simulink subsystem "accelerometer"  (R2024b)
settings: Solver=VariableStepAuto  StartTime=0.0  StopTime=10.0  RelTol=1e-3
undefined symbols (not defined in the file or in its folder): ACCEL_BIAS, ACCEL_COV, ACCEL_RANGE, ACCEL_RATE
settings Model: Creator=yevge  LastModifiedBy=Aiden Gaydos

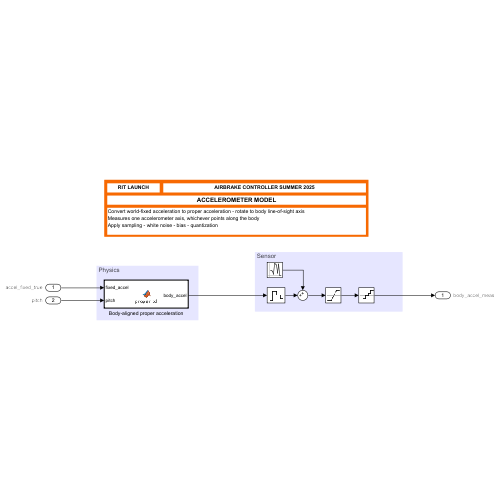
[thumbnail: Simulink's stored preview of the top-level diagram]
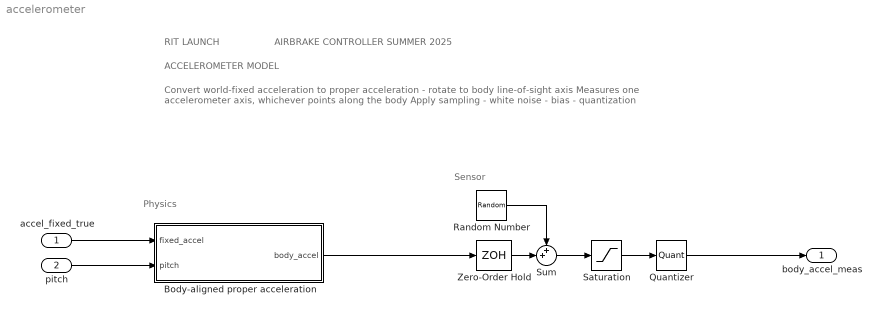
== system accelerometer ==
  note: Sensor
  note: Physics
  note: AIRBRAKE CONTROLLER SUMMER 2025
  note: RIT LAUNCH
  note: ACCELEROMETER MODEL
  note: Convert world-fixed acceleration to proper acceleration - rotate to body line-of-sight axis
      | Measures one accelerometer axis, whichever points along the body
      | Apply sampling - white noise - bias - quantization
  accel_fixed_true : Inport  Unit=m/s^2  PortDimensions=[2 1]
  pitch : Inport  Port=2  Unit=rad  PortDimensions=1
  Body-aligned proper acceleration : MATLAB Function  TreatAsAtomicUnit=on
  Quantizer : Quantizer  QuantizationInterval=ACCEL_LSB
  Random Number : RandomNumber  Mean=ACCEL_BIAS  Variance=ACCEL_COV  SampleTime=1/ACCEL_RATE
  Saturation : Saturate  UpperLimit=ACCEL_RANGE  LowerLimit=-ACCEL_RANGE
  Sum : Sum  Inputs=++|
  Zero-Order Hold : ZeroOrderHold  SampleTime=1/ACCEL_RATE
  body_accel_meas : Outport  Unit=m/s^2  PortDimensions=1
  wires:
  pitch/1 -> Body-aligned proper acceleration/2(pitch)
  Sum/1 -> Saturation/1
  Quantizer/1 -> body_accel_meas/1
  Random Number/1 -> Sum/1
  accel_fixed_true/1 -> Body-aligned proper acceleration/1(fixed_accel)
  Body-aligned proper acceleration/1(body_accel) -> Zero-Order Hold/1
  Zero-Order Hold/1 -> Sum/2
  Saturation/1 -> Quantizer/1

== matlab function accelerometer/Body-aligned proper acceleration ==
  data: fixed_accel input; pitch input size=1; body_accel output size=1; GRAVITY parameter
function body_accel = proper_xl(fixed_accel, pitch, GRAVITY)
    proper_accel = fixed_accel + [0; GRAVITY];
    % dot(proper accel, body LOS) is body aligned proper acceleration
    body_accel = cos(pitch) * proper_accel(1) + sin(pitch) * proper_accel(2);
end
